simulink model "model2_diss"  (R2021b)
settings: Solver=VariableStepAuto  StartTime=0.0  StopTime=10  RelTol=1e-3
InitFcn:
  | %param;
values from neighbouring files (symbols this model uses):
  P =     [P.mat]    (also in expand_path_points.m = P1 *(1 - t) + t * P2)
undefined symbols (not defined in the file or in its folder): autopilot, forces_moments, true_states
libraries: simulink x3
settings Model: Creator=hpShe  LastModifiedBy=hpShe

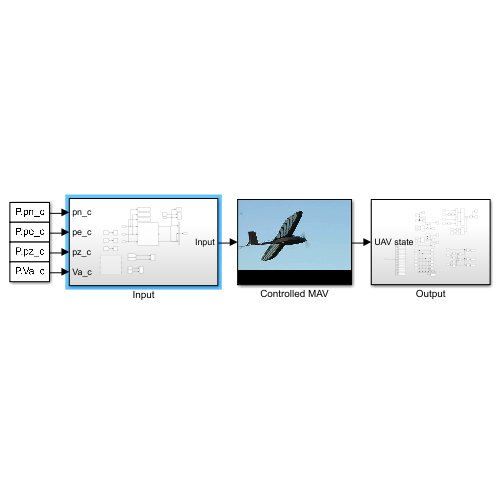
[thumbnail: Simulink's stored preview of the top-level diagram]
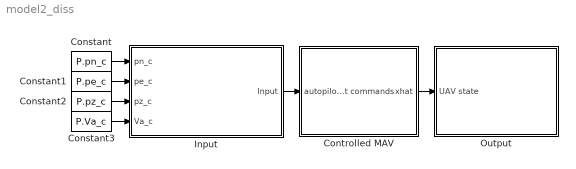
== system model2_diss ==
  Constant : Constant  Value=P.pn_c
  Constant1 : Constant  Value=P.pe_c
  Constant2 : Constant  Value=P.pz_c
  Constant3 : Constant  Value=P.Va_c
  Controlled MAV : Subsystem
      mask Display: image(imread('batcam.png'))
  Input : Subsystem
  Output : Subsystem
  wires:
  Controlled MAV/1(xhat) -> Output/1(UAV state)
  Input/1(Input) -> Controlled MAV/1(autopilot commands)
  Constant/1 -> Input/1(pn_c)
  Constant1/1 -> Input/2(pe_c)
  Constant2/1 -> Input/3(pz_c)
  Constant3/1 -> Input/4(Va_c)

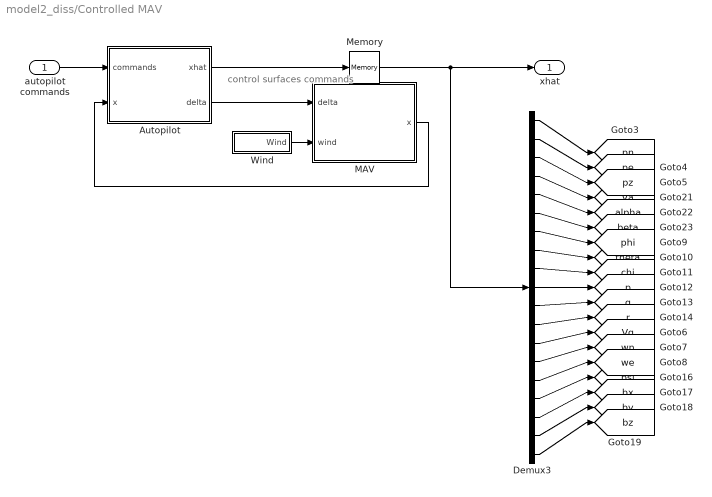
== system model2_diss/Controlled MAV ==
  note: control surfaces
      | commands
  autopilot commands : Inport
  Autopilot : Subsystem
      mask Display: image(imread('kestrel.jpg'))
  Demux3 : Demux  Outputs=19
  MAV : Subsystem
      mask Display: image(imread('batcam.png'))
  Memory : Memory
  Wind : Subsystem
  xhat : Outport
  tag scope: Va=global, Vg=global, alpha=global, beta=global, bx=global, by=global, bz=global, chi=global, p=global, pe=global, phi=global, pn=global, psi=global, pz=global, q=global, r=global, theta=global, we=global, wn=global
  wires:
  MAV/1(x) -> Autopilot/2(x)
  Autopilot/1(xhat) -> Memory/1
  autopilot commands/1 -> Autopilot/1(commands)
  Autopilot/2(delta) -> MAV/1(delta)
  Wind/1(Wind) -> MAV/2(wind)
  Demux3/16 -> [psi]
  Demux3/14 -> [wn]
  Demux3/13 -> [Vg]
  Demux3/10 -> [p]
  Demux3/15 -> [we]
  Demux3/2 -> [pe]
  Demux3/5 -> [alpha]
  Demux3/18 -> [by]
  Demux3/8 -> [theta]
  Demux3/12 -> [r]
  Demux3/1 -> [pn]
  Demux3/3 -> [pz]
  Demux3/9 -> [chi]
  Demux3/17 -> [bx]
  Memory/1 -> xhat/1, Demux3/1
  Demux3/7 -> [phi]
  Demux3/19 -> [bz]
  Demux3/4 -> [Va]
  Demux3/6 -> [beta]
  Demux3/11 -> [q]

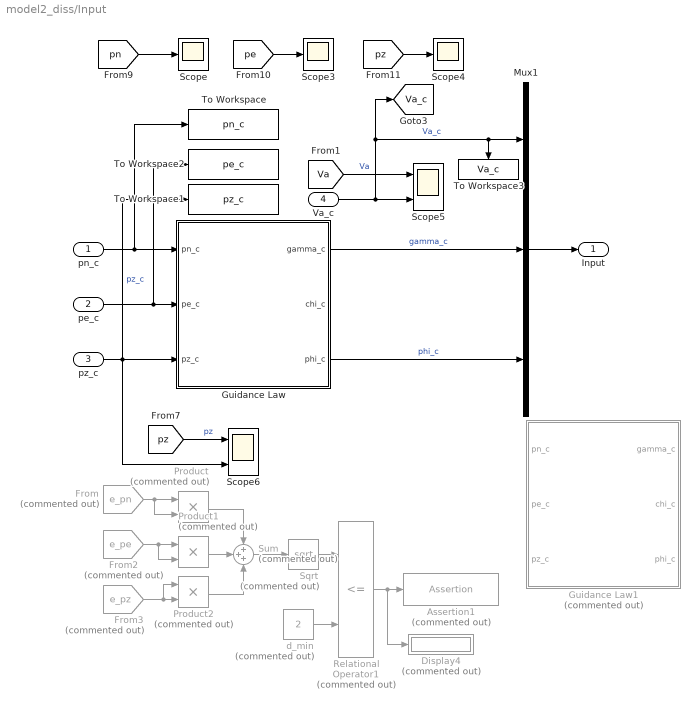
== system model2_diss/Input ==
  pn_c : Inport
  pe_c : Inport  Port=2
  pz_c : Inport  Port=3
  Va_c : Inport  Port=4
  Assertion1 : Assertion  Commented=on  AssertionFailFcn=set_param(bdroot,'SimulationCommand','stop');  StopWhenAssertionFail=off
  Display4 : Display  Commented=on
  From : From  Commented=on  GotoTag=e_pn  TagVisibility=global
  From2 : From  Commented=on  GotoTag=e_pe  TagVisibility=global
  From3 : From  Commented=on  GotoTag=e_pz  TagVisibility=global
  Guidance Law : Subsystem
  Guidance Law1 : Subsystem  Commented=on
  Mux1 : Mux  Inputs=3
  Product : Product  Commented=on
  Product1 : Product  Commented=on
  Product2 : Product  Commented=on
  Relational Operator1 : RelationalOperator  Commented=on  Operator=<=  OutDataTypeStr=boolean  RndMeth=Simplest
  Scope : Scope
  Scope3 : Scope
  Scope4 : Scope
  Scope5 : Scope  NumInputPorts=2
  Scope6 : Scope  NumInputPorts=2
  Sqrt : Sqrt  Commented=on  SaturateOnIntegerOverflow=on
  Sum : Sum  Commented=on  Inputs=+++
  To Workspace : ToWorkspace  VariableName=pn_c  SaveFormat=Timeseries  SampleTime=-1
  To Workspace1 : ToWorkspace  VariableName=pz_c  SaveFormat=Timeseries  SampleTime=-1
  To Workspace2 : ToWorkspace  VariableName=pe_c  SaveFormat=Timeseries  SampleTime=-1
  To Workspace3 : ToWorkspace  VariableName=Va_c  SaveFormat=Timeseries  SampleTime=-1
  d_min : Constant  Commented=on  Value=2
  Input : Outport
  tag scope: Va_c=global
  wires:
  [Va] -> Scope5/1  "Va"
  Va_c/1 -> To Workspace3/1, Mux1/1, [Va_c], Scope5/2  "Va_c"
  [pn] -> Scope/1
  [pe] -> Scope3/1
  [pz] -> Scope4/1
  pe_c/1 -> Guidance Law/2(pe_c), To Workspace2/1
  pn_c/1 -> Guidance Law/1(pn_c), To Workspace/1
  Mux1/1 -> Input/1
  Guidance Law/1(gamma_c) -> Mux1/2  "gamma_c"
  Guidance Law/3(phi_c) -> Mux1/3  "phi_c"
  [pz] -> Scope6/1  "pz"
  pz_c/1 -> Guidance Law/3(pz_c), Scope6/2, To Workspace1/1  "pz_c"
  Relational Operator1/1 -> Display4/1, Assertion1/1
  Sqrt/1 -> Relational Operator1/1
  Sum/1 -> Sqrt/1
  Product1/1 -> Sum/2
  From/1 -> Product/1, Product/2
  From2/1 -> Product1/2, Product1/1
  From3/1 -> Product2/1, Product2/2
  d_min/1 -> Relational Operator1/2
  Product/1 -> Sum/1
  Product2/1 -> Sum/3

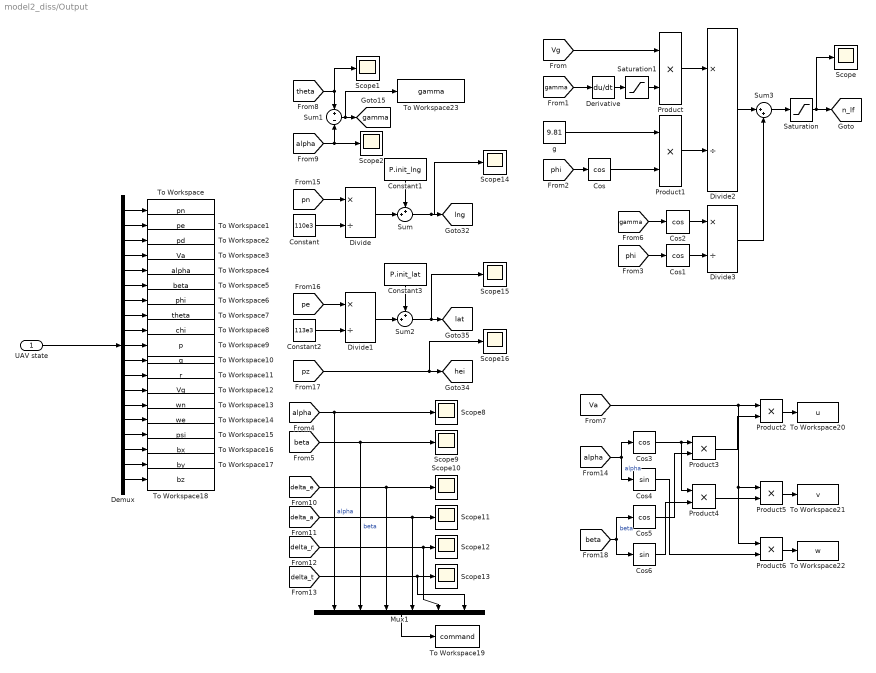
== system model2_diss/Output ==
  UAV state : Inport
  Constant : Constant  Value=110e3
  Constant1 : Constant  Value=P.init_lng
  Constant2 : Constant  Value=113e3
  Constant3 : Constant  Value=P.init_lat
  Cos{,1..3,5} (5 alike) : Trigonometry  Operator=cos
  Cos4 : Trigonometry
  Cos6 : Trigonometry
  Demux : Demux  Outputs=19
  Derivative : Derivative
  Divide{,1..3} (4 alike) : Product  Inputs=*/
  Mux1 : Mux  Inputs=6
  Product{,1..6} (7 alike) : Product
  Saturation : Saturate  UpperLimit=2.1  LowerLimit=0
  Saturation1 : Saturate  UpperLimit=5  LowerLimit=-5
  Scope{,1..2,8..16} (12 alike) : Scope
  Sum : Sum  Inputs=++|
  Sum1 : Sum  Inputs=+-
  Sum2 : Sum  Inputs=++|
  Sum3 : Sum  Inputs=|++
  To Workspace : ToWorkspace  VariableName=pn  SaveFormat=Timeseries  SampleTime=-1
  To Workspace1 : ToWorkspace  VariableName=pe  SaveFormat=Timeseries  SampleTime=-1
  To Workspace10 : ToWorkspace  VariableName=q  SaveFormat=Timeseries  SampleTime=-1
  To Workspace11 : ToWorkspace  VariableName=r  SaveFormat=Timeseries  SampleTime=-1
  To Workspace12 : ToWorkspace  VariableName=Vg  SaveFormat=Timeseries  SampleTime=-1
  To Workspace13 : ToWorkspace  VariableName=wn  SaveFormat=Timeseries  SampleTime=-1
  To Workspace14 : ToWorkspace  VariableName=we  SaveFormat=Timeseries  SampleTime=-1
  To Workspace15 : ToWorkspace  VariableName=psi  SaveFormat=Timeseries  SampleTime=-1
  To Workspace16 : ToWorkspace  VariableName=bx  SaveFormat=Timeseries  SampleTime=-1
  To Workspace17 : ToWorkspace  VariableName=by  SaveFormat=Timeseries  SampleTime=-1
  To Workspace18 : ToWorkspace  VariableName=bz  SaveFormat=Timeseries  SampleTime=-1
  To Workspace19 : ToWorkspace  VariableName=command  SaveFormat=Timeseries  SampleTime=-1
  To Workspace2 : ToWorkspace  VariableName=pd  SaveFormat=Timeseries  SampleTime=-1
  To Workspace20 : ToWorkspace  VariableName=u  SaveFormat=Timeseries  SampleTime=-1
  To Workspace21 : ToWorkspace  VariableName=v  SaveFormat=Timeseries  SampleTime=-1
  To Workspace22 : ToWorkspace  VariableName=w  SaveFormat=Timeseries  SampleTime=-1
  To Workspace23 : ToWorkspace  VariableName=gamma  SaveFormat=Timeseries  SampleTime=-1
  To Workspace3 : ToWorkspace  VariableName=Va  SaveFormat=Timeseries  SampleTime=-1
  To Workspace4 : ToWorkspace  VariableName=alpha  SaveFormat=Timeseries  SampleTime=-1
  To Workspace5 : ToWorkspace  VariableName=beta  SaveFormat=Timeseries  SampleTime=-1
  To Workspace6 : ToWorkspace  VariableName=phi  SaveFormat=Timeseries  SampleTime=-1
  To Workspace7 : ToWorkspace  VariableName=theta  SaveFormat=Timeseries  SampleTime=-1
  To Workspace8 : ToWorkspace  VariableName=chi  SaveFormat=Timeseries  SampleTime=-1
  To Workspace9 : ToWorkspace  VariableName=p  SaveFormat=Timeseries  SampleTime=-1
  g : Constant  Value=9.81
  tag scope: gamma=global, hei=global, lat=global, lng=global, n_lf=global
  wires:
  Demux/15 -> To Workspace14/1
  Demux/13 -> To Workspace12/1
  Demux/4 -> To Workspace3/1
  Demux/19 -> To Workspace18/1
  Sum/1 -> Scope14/1, [lng]
  [pz] -> Scope16/1, [hei]
  Demux/8 -> To Workspace7/1
  Demux/7 -> To Workspace6/1
  Constant2/1 -> Divide1/2
  Demux/17 -> To Workspace16/1
  Demux/3 -> To Workspace2/1
  Sum2/1 -> Scope15/1, [lat]
  Demux/11 -> To Workspace10/1
  Divide/1 -> Sum/2
  UAV state/1 -> Demux/1
  Demux/18 -> To Workspace17/1
  [alpha] -> Scope2/1, Sum1/2
  Demux/5 -> To Workspace4/1
  Demux/12 -> To Workspace11/1
  Demux/2 -> To Workspace1/1
  Demux/10 -> To Workspace9/1
  Constant1/1 -> Sum/1
  Demux/1 -> To Workspace/1
  Demux/6 -> To Workspace5/1
  Demux/16 -> To Workspace15/1
  Constant3/1 -> Sum2/1
  Demux/9 -> To Workspace8/1
  Demux/14 -> To Workspace13/1
  [theta] -> Sum1/1, Scope1/1
  [pe] -> Divide1/1
  [pn] -> Divide/1
  Divide1/1 -> Sum2/2
  Constant/1 -> Divide/2
  Sum1/1 -> To Workspace23/1, [gamma]
  [alpha] -> Mux1/1, Scope8/1  "alpha"
  [delta_e] -> Scope10/1, Mux1/3
  [delta_a] -> Scope11/1, Mux1/4
  Mux1/1 -> To Workspace19/1
  [beta] -> Scope9/1, Mux1/2  "beta"
  [delta_r] -> Scope12/1, Mux1/5
  [delta_t] -> Scope13/1, Mux1/6
  [gamma] -> Derivative/1
  [Vg] -> Product/1
  Product/1 -> Divide2/1
  Product1/1 -> Divide2/2
  g/1 -> Product1/1
  [phi] -> Cos/1
  Cos/1 -> Product1/2
  Divide2/1 -> Sum3/1
  Divide3/1 -> Sum3/2
  Cos1/1 -> Divide3/2
  [phi] -> Cos1/1
  [gamma] -> Cos2/1
  Cos2/1 -> Divide3/1
  Sum3/1 -> Saturation/1
  Saturation/1 -> Scope/1, [n_lf]
  Derivative/1 -> Saturation1/1
  Saturation1/1 -> Product/2
  [Va] -> Product5/1, Product6/1, Product2/1
  [alpha] -> Cos3/1, Cos4/1  "alpha"
  [beta] -> Cos6/1, Cos5/1  "beta"
  Cos3/1 -> Product4/1, Product3/1
  Cos5/1 -> Product3/2
  Product3/1 -> Product2/2
  Product2/1 -> To Workspace20/1
  Cos6/1 -> Product4/2
  Product4/1 -> Product5/2
  Product5/1 -> To Workspace21/1
  Product6/1 -> To Workspace22/1
  Cos4/1 -> Product6/2

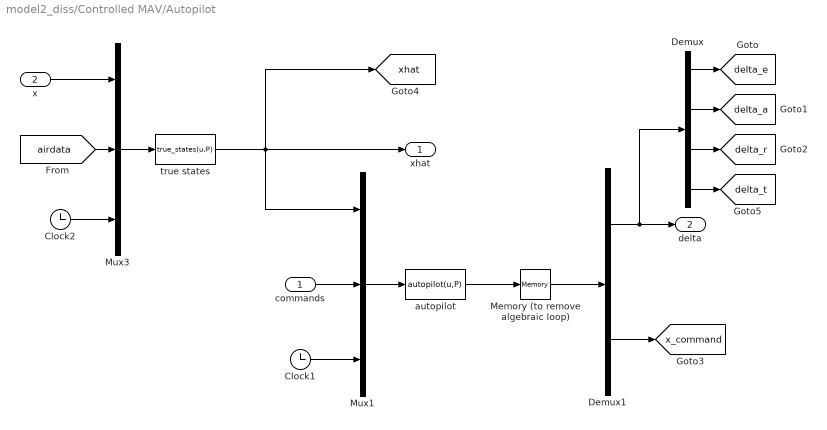
== system model2_diss/Controlled MAV/Autopilot ==
  commands : Inport
  x : Inport  Port=2
  Clock1 : Clock
  Clock2 : Clock
  Demux : Demux
  Demux1 : Demux  Outputs=[4;12]
  Memory (to remove algebraic loop) : Memory
  Mux1 : Mux  Inputs=3
  Mux3 : Mux  Inputs=3
  autopilot : MATLABFcn  MATLABFcn=autopilot(u,P)  OutputDimensions=4+12  SampleTime=P.Ts
  true states : MATLABFcn  MATLABFcn=true_states(u,P)  OutputDimensions=19  SampleTime=P.Ts
  xhat : Outport
  delta : Outport  Port=2
  tag scope: delta_a=global, delta_e=global, delta_r=global, delta_t=global, x_command=global, xhat=global
  wires:
  Memory (to remove algebraic loop)/1 -> Demux1/1
  Clock2/1 -> Mux3/3
  Clock1/1 -> Mux1/3
  x/1 -> Mux3/1
  [airdata] -> Mux3/2
  Mux3/1 -> true states/1
  true states/1 -> xhat/1, Mux1/1, [xhat]
  commands/1 -> Mux1/2
  Demux1/2 -> [x_command]
  Demux1/1 -> Demux/1, delta/1
  autopilot/1 -> Memory (to remove algebraic loop)/1
  Mux1/1 -> autopilot/1
  Demux/1 -> [delta_e]
  Demux/2 -> [delta_a]
  Demux/3 -> [delta_r]
  Demux/4 -> [delta_t]

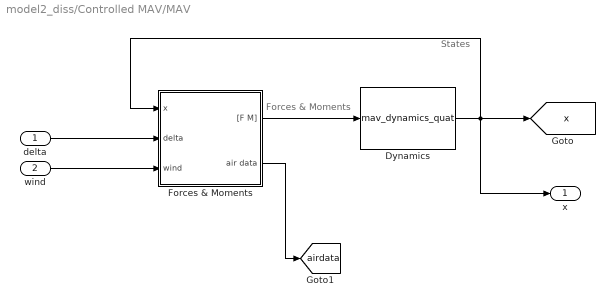
== system model2_diss/Controlled MAV/MAV ==
  note: States
  note: Forces & Moments
  delta : Inport
  wind : Inport  Port=2
  Dynamics : S-Function  FunctionName=mav_dynamics_quat  Parameters=mass,Jx,Jy,Jz,Jxz,pn0,pe0,pd0,u0,v0,w0,phi0,theta0,psi0,p0,q0,r0  SFunctionDeploymentMode=off  EnableBusSupport=off  mask{mass=P.mass, Jx=P.Jx, Jy=P.Jy, Jz=P.Jz, Jxz=P.Jxz, pn0=P.pn0, pe0=P.pe0, pd0=P.pd0, u0=P.u0, v0=P.v0, w0=P.w0, phi0=P.phi0, theta0=P.theta0, psi0=P.psi0, p0=P.p0, q0=P.q0, r0=P.r0}
      mask prompts: pn0 "Initial North position"; pe0 "Initial East position"; pd0 "Initial Down position"; u0 "Initial velocy u0"; v0 "Initial velocity v0"; w0 "Initial velocity w0"; phi0 "Initial roll angle"; theta0 "Initial pitch angle"; psi0 "Initial yaw angle"; p0 "Initial roll rate"; q0 "Initial pitch rate"; r0 "Initial yaw rate"
  Forces & Moments : Subsystem
  x : Outport
  tag scope: airdata=global, x=global
  wires:
  wind/1 -> Forces & Moments/3(wind)
  delta/1 -> Forces & Moments/2(delta)
  Forces & Moments/2(air data) -> [airdata]
  Forces & Moments/1("[F M]") -> Dynamics/1
  Dynamics/1 -> [x], Forces & Moments/1(x), x/1

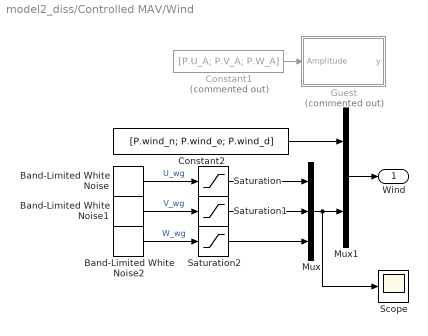
== system model2_diss/Controlled MAV/Wind ==
  Band-Limited White Noise : simulink/Sources/Band-Limited White Noise  Cov=0.1  Ts=0.1  seed=[23341]
  Band-Limited White Noise1 : simulink/Sources/Band-Limited White Noise  Cov=0.1  Ts=0.1  seed=[23341]
  Band-Limited White Noise2 : simulink/Sources/Band-Limited White Noise  Cov=0.1  Ts=0.1  seed=[23341]
  Constant1 : Constant  Commented=on  Value=[P.U_A; P.V_A; P.W_A]
  Constant2 : Constant  Value=[P.wind_n; P.wind_e; P.wind_d]
  Guest : MATLAB Function  Commented=on  TreatAsAtomicUnit=on
  Mux : Mux  Inputs=3
  Mux1 : Mux  Inputs=2
  Saturation : Saturate  UpperLimit=P.U_A  LowerLimit=-P.U_A
  Saturation1 : Saturate  UpperLimit=P.V_A  LowerLimit=-P.V_A
  Saturation2 : Saturate  UpperLimit=P.W_A  LowerLimit=-P.W_A
  Scope : Scope
  Wind : Outport
  wires:
  Mux1/1 -> Wind/1
  Constant2/1 -> Mux1/1
  Constant1/1 -> Guest/1(Amplitude)
  Mux/1 -> Scope/1, Mux1/2
  Band-Limited White Noise1/1 -> Saturation1/1  "V_wg"
  Band-Limited White Noise2/1 -> Saturation2/1  "W_wg"
  Saturation/1 -> Mux/1
  Band-Limited White Noise/1 -> Saturation/1  "U_wg"
  Saturation1/1 -> Mux/2
  Saturation2/1 -> Mux/3

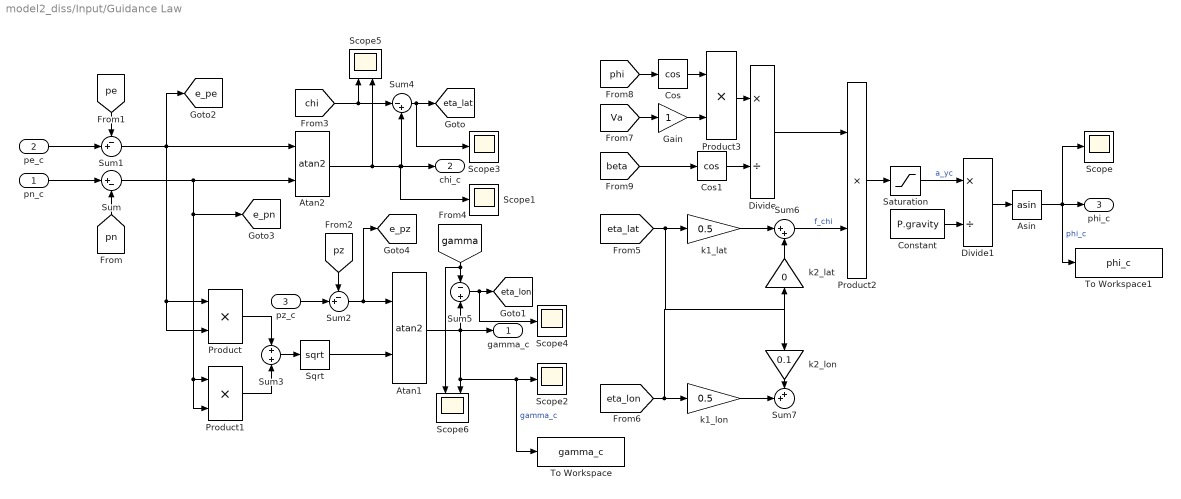
== system model2_diss/Input/Guidance Law ==
  pn_c : Inport
  pe_c : Inport  Port=2
  pz_c : Inport  Port=3
  Asin : Trigonometry  Operator=asin
  Atan1 : Trigonometry  Operator=atan2
  Atan2 : Trigonometry  Operator=atan2
  Constant : Constant  Value=P.gravity
  Cos : Trigonometry  Operator=cos
  Cos1 : Trigonometry  Operator=cos
  Divide : Product  Inputs=*/
  Divide1 : Product  Inputs=*/
  Gain : Gain
  Product{,1..3} (4 alike) : Product
  Saturation : Saturate  UpperLimit=P.gravity  LowerLimit=-P.gravity
  Scope{,1..4} (5 alike) : Scope
  Scope5 : Scope  NumInputPorts=2
  Scope6 : Scope  NumInputPorts=2
  Sqrt : Sqrt  SaturateOnIntegerOverflow=on
  Sum : Sum  Inputs=|+-
  Sum1 : Sum  Inputs=-+|
  Sum2 : Sum  Inputs=-+|
  Sum3 : Sum
  Sum4 : Sum  Inputs=|-+
  Sum5 : Sum  Inputs=-+
  Sum6 : Sum  Inputs=|++
  Sum7 : Sum  Inputs=++|
  To Workspace : ToWorkspace  VariableName=gamma_c  SaveFormat=Timeseries  SampleTime=-1
  To Workspace1 : ToWorkspace  VariableName=phi_c  SaveFormat=Timeseries  SampleTime=-1
  k1_lat : Gain  Gain=0.5
  k1_lon : Gain  Gain=0.5
  k2_lat : Gain  Gain=0
  k2_lon : Gain  Gain=0.1
  gamma_c : Outport
  chi_c : Outport  Port=2
  phi_c : Outport  Port=3
  tag scope: e_pe=global, e_pn=global, e_pz=global, eta_lat=global, eta_lon=global
  wires:
  pe_c/1 -> Sum1/2
  pz_c/1 -> Sum2/2
  [pe] -> Sum1/1
  [pz] -> Sum2/1
  Sum1/1 -> [e_pe], Product/2, Product/1, Atan2/1
  pn_c/1 -> Sum/1
  [pn] -> Sum/2
  Sum/1 -> [e_pn], Product1/2, Product1/1, Atan2/2
  Atan2/1 -> Scope5/2, Sum4/2, chi_c/1, Scope1/1
  Product/1 -> Sum3/1
  Product1/1 -> Sum3/2
  Sum3/1 -> Sqrt/1
  Sum2/1 -> [e_pz], Atan1/1
  Sqrt/1 -> Atan1/2
  Atan1/1 -> gamma_c/1, Scope6/2, To Workspace/1, Scope2/1, Sum5/2  "gamma_c"
  [chi] -> Scope5/1, Sum4/1
  Sum4/1 -> Scope3/1, [eta_lat]
  [gamma] -> Scope6/1, Sum5/1
  Sum5/1 -> Scope4/1, [eta_lon]
  [eta_lat] -> k1_lat/1, k2_lon/1
  [eta_lon] -> k2_lat/1, k1_lon/1
  k1_lat/1 -> Sum6/1
  k2_lat/1 -> Sum6/2
  k1_lon/1 -> Sum7/2
  k2_lon/1 -> Sum7/1
  Sum6/1 -> Product2/2  "f_chi"
  [Va] -> Gain/1
  Gain/1 -> Product3/2
  [phi] -> Cos/1
  Cos/1 -> Product3/1
  Product3/1 -> Divide/1
  Cos1/1 -> Divide/2
  [beta] -> Cos1/1
  Divide/1 -> Product2/1
  Product2/1 -> Saturation/1
  Saturation/1 -> Divide1/1  "a_yc"
  Constant/1 -> Divide1/2
  Divide1/1 -> Asin/1
  Asin/1 -> To Workspace1/1, Scope/1, phi_c/1  "phi_c"

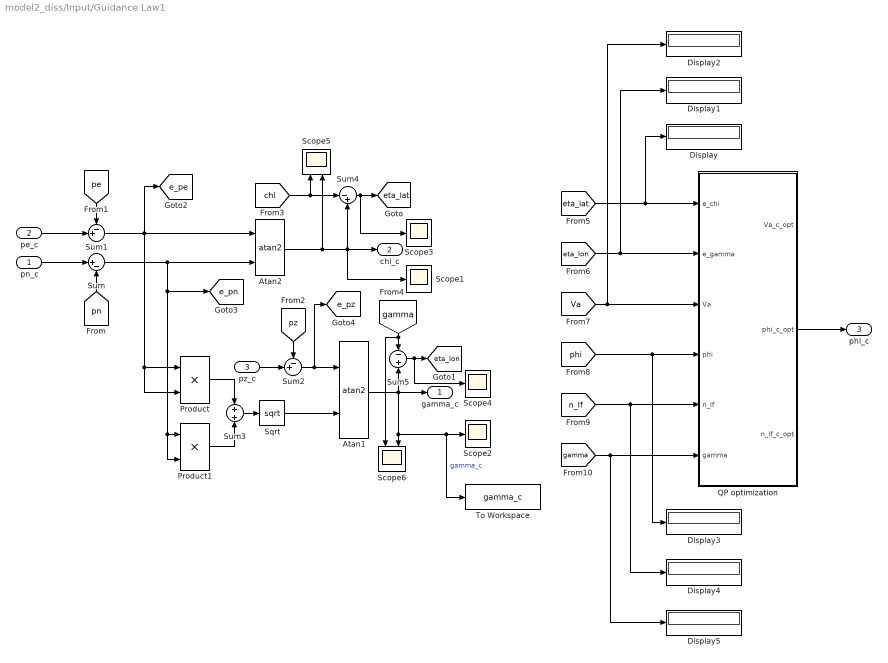
== system model2_diss/Input/Guidance Law1 ==
  pn_c : Inport
  pe_c : Inport  Port=2
  pz_c : Inport  Port=3
  Atan1 : Trigonometry  Operator=atan2
  Atan2 : Trigonometry  Operator=atan2
  Display{,1..5} (6 alike) : Display
  Product : Product
  Product1 : Product
  QP optimization : MATLAB Function  TreatAsAtomicUnit=on
  Scope{1..4} (4 alike) : Scope
  Scope5 : Scope  NumInputPorts=2
  Scope6 : Scope  NumInputPorts=2
  Sqrt : Sqrt  SaturateOnIntegerOverflow=on
  Sum : Sum  Inputs=|+-
  Sum1 : Sum  Inputs=-+|
  Sum2 : Sum  Inputs=-+|
  Sum3 : Sum
  Sum4 : Sum  Inputs=|-+
  Sum5 : Sum  Inputs=-+
  To Workspace : ToWorkspace  VariableName=gamma_c  SaveFormat=Timeseries  SampleTime=-1
  gamma_c : Outport
  chi_c : Outport  Port=2
  phi_c : Outport  Port=3
  tag scope: e_pe=global, e_pn=global, e_pz=global, eta_lat=global, eta_lon=global
  wires:
  pe_c/1 -> Sum1/2
  pz_c/1 -> Sum2/2
  [pe] -> Sum1/1
  [pz] -> Sum2/1
  Sum1/1 -> [e_pe], Product/2, Product/1, Atan2/1
  pn_c/1 -> Sum/1
  [pn] -> Sum/2
  Sum/1 -> [e_pn], Product1/2, Product1/1, Atan2/2
  Atan2/1 -> Scope5/2, Sum4/2, chi_c/1, Scope1/1
  Product/1 -> Sum3/1
  Product1/1 -> Sum3/2
  Sum3/1 -> Sqrt/1
  Sum2/1 -> [e_pz], Atan1/1
  Sqrt/1 -> Atan1/2
  Atan1/1 -> gamma_c/1, Scope6/2, To Workspace/1, Scope2/1, Sum5/2  "gamma_c"
  [chi] -> Scope5/1, Sum4/1
  Sum4/1 -> Scope3/1, [eta_lat]
  [gamma] -> Scope6/1, Sum5/1
  Sum5/1 -> Scope4/1, [eta_lon]
  [eta_lat] -> Display/1, QP optimization/1(e_chi)
  [eta_lon] -> Display1/1, QP optimization/2(e_gamma)
  [Va] -> Display2/1, QP optimization/3(Va)
  [phi] -> Display3/1, QP optimization/4(phi)
  [n_lf] -> Display4/1, QP optimization/5(n_lf)
  [gamma] -> Display5/1, QP optimization/6(gamma)
  QP optimization/2(phi_c_opt) -> phi_c/1

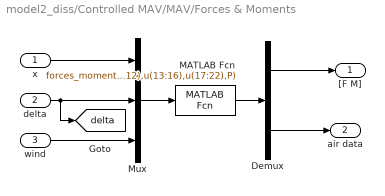
== system model2_diss/Controlled MAV/MAV/Forces & Moments ==
  x : Inport
  delta : Inport  Port=2
  wind : Inport  Port=3
  Demux : Demux  Outputs=[6;6]
  MATLAB Fcn : MATLABFcn  MATLABFcn=forces_moments(u(1:12),u(13:16),u(17:22),P)  OutputDimensions=12
  Mux : Mux  Inputs=3
  "[F M]" : Outport
  air data : Outport  Port=2
  tag scope: delta=global
  wires:
  x/1 -> Mux/1
  delta/1 -> Mux/2, [delta]
  wind/1 -> Mux/3
  MATLAB Fcn/1 -> Demux/1
  Demux/1 -> "[F M]"/1
  Mux/1 -> MATLAB Fcn/1
  Demux/2 -> air data/1

== matlab function model2_diss/Input/Guidance Law1/QP optimization ==
  data: e_chi input; e_gamma input; Va input; Va_c_opt output; phi input; n_lf input; gamma input; phi_c_opt output; n_lf_c_opt output
function [Va_c_opt,phi_c_opt,n_lf_c_opt] = QP_optimization(e_chi,e_gamma,Va,phi,n_lf,gamma)
    
    g = 9.81;
    b_Va = 0.5;
    b_phi = 0.1;
    b_n_lf = 0.25;
    epsilon_star = 1.5;

    u_max = [16, 0.6, 2.1]';
    u_min = [9, -0.6, 0]';
    R = diag([0.02, 1, 1]);

    f = [g/Va * tan(phi);... 
         g/Va * (n_lf * cos(phi) - cos(gamma));...
         -b_Va * Va;...
         -b_phi * phi;...
         -b_n_lf * n_lf];
    g = [zeros(2,3);diag([b_Va,b_phi,b_n_lf])];

    Lambda = [eye(2),zeros(2,3)];

    F = - Lambda * f;
    G = - Lambda * g;

    e = [e_chi; e_gamma];

    A = e' * G;
    b = -e' * (F + epsilon_star/2 * e);

    x0 = [9,0,1];
    options = optimoptions('quadprog','Algorithm','active-set');
    
    u_opt = quadprog(R,zeros(3,1),A,b,[],[],u_min,u_max,x0,options);

    Va_c_opt = u_opt(1);
    phi_c_opt = u_opt(2);
    n_lf_c_opt = u_opt(3);
end

== matlab function model2_diss/Controlled MAV/Wind/Guest ==
  data: Amplitude input; y output
function y = Guest(Amplitude)
  U_A = Amplitude(1);
  V_A = Amplitude(2);
  W_A = Amplitude(3);
  
  U_wg = 2 * U_A * rand() - U_A;
  V_wg = 2 * V_A * rand() - V_A;
  W_wg = 2 * W_A * rand() - W_A;

  y = [U_wg;V_wg;W_wg];

end
